simulink model "UAV_2010_simulink_model_run"  (R2022b)
settings: Solver=VariableStepAuto  StartTime=0.0  StopTime=t_end  RelTol=1e-3
values from neighbouring files (symbols this model uses):
  alt0 = 500    [Run_nonlinear_2010UAV_sim.m]
  lat0 = deg2rad(63.9963)    [Run_nonlinear_2010UAV_sim.m]
  long0 = deg2rad(-22.6237)    [Run_nonlinear_2010UAV_sim.m]
  windseed = [randi([0 4000], 1, 4)]    [Run_nonlinear_2010UAV_sim.m]
  X_init = X_trim_point    [Run_nonlinear_2010UAV_sim.m]
undefined symbols (not defined in the file or in its folder): F, Light, MIL, Receive, Send
libraries: aerolibfltsims x4, aerolibwind2 x2, aerolibatmos2 x1
settings Model: Creator=aaron  LastModifiedBy=aaron
settings DataIOCC: SaveFormat=StructureWithTime
settings DebuggingCC: UnderSpecifiedDimensionMsg=warning

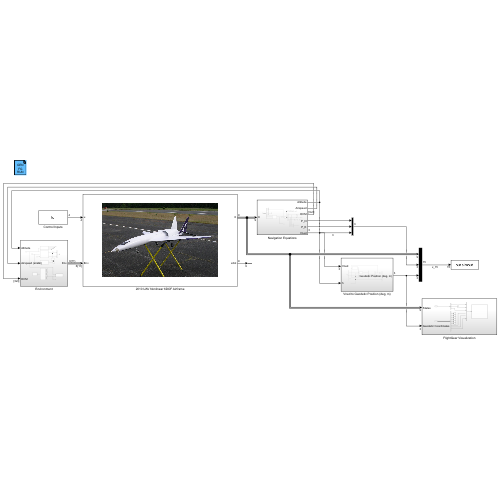
[thumbnail: Simulink's stored preview of the top-level diagram]
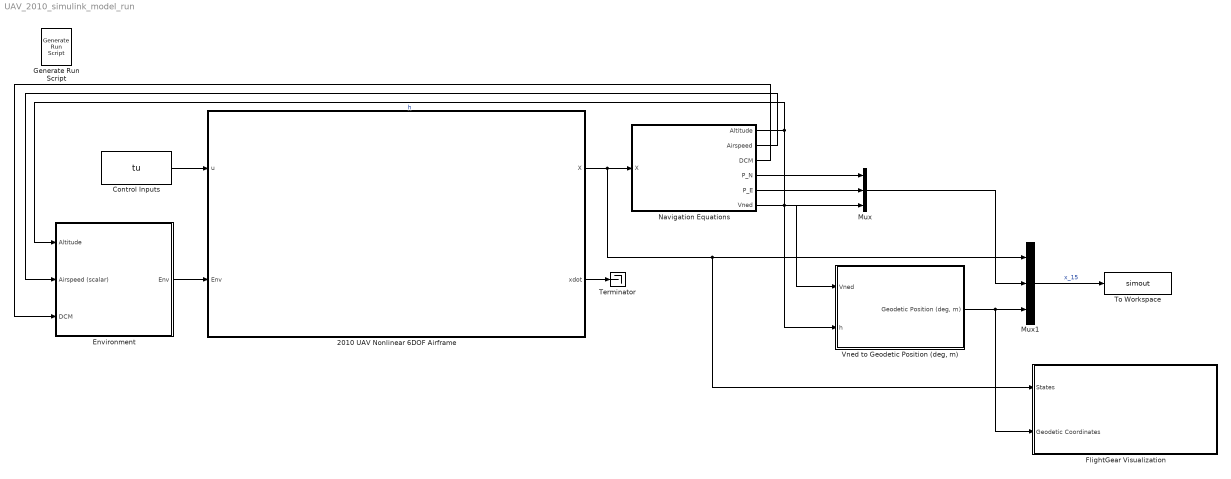
== system UAV_2010_simulink_model_run ==
  2010 UAV Nonlinear 6DOF Airframe : Subsystem
      mask Display: image('$imagefile'); % Use "Edit Image" on toolstrip to change.
  Control Inputs : FromWorkspace  VariableName=tu
  Environment : Subsystem
  FlightGear Visualization : Subsystem
  Generate Run Script : aerolibfltsims/Generate Run Script  Architecture=Default  dataFlow=Send-Receive  GeometryModelName=c172p  AirportId=KSFO  RunwayId=10L  InitialAltitude=7224  InitialHeading=113  OffsetDistance=4.72  OffsetAzimuth=0  InstallScenery=off  DisableShaders=on  OriginAddress=127.0.0.1  DestinationPort=5502  OriginPort=5505  LocalAddress=127.0.0.1  OutputFileName=fg_simulink_2010UAV.bat  FlightGearBaseDirectory=C:\Program Files\FlightGear 2020.3
  Mux : Mux  Inputs=3
  Mux1 : Mux  Inputs=[9 3 3]
  Navigation Equations : Subsystem
  Terminator : Terminator
  To Workspace : ToWorkspace  VariableName=simout  SaveFormat=Structure With Time  SampleTime=-1
  "Vned to Geodetic Position (deg, m)" : Subsystem
  wires:
  Control Inputs/1 -> 2010 UAV Nonlinear 6DOF Airframe/1(u)
  2010 UAV Nonlinear 6DOF Airframe/2(xdot) -> Terminator/1
  2010 UAV Nonlinear 6DOF Airframe/1(X) -> Navigation Equations/1(X), FlightGear Visualization/1(States), Mux1/1
  Navigation Equations/4(P_N) -> Mux/1
  Navigation Equations/5(P_E) -> Mux/2
  Navigation Equations/1(Altitude) -> Mux/3, "Vned to Geodetic Position (deg, m)"/2(h), Environment/1(Altitude)  "h"
  Navigation Equations/3(DCM) -> Environment/3(DCM)
  Mux/1 -> Mux1/2
  Mux1/1 -> To Workspace/1  "x_15"
  Navigation Equations/2(Airspeed) -> Environment/2(Airspeed (scalar))
  Navigation Equations/6(Vned) -> "Vned to Geodetic Position (deg, m)"/1(Vned)
  "Vned to Geodetic Position (deg, m)"/1("Geodetic Position (deg, m)") -> FlightGear Visualization/2(Geodetic Coordinates), Mux1/3
  Environment/1(Env) -> 2010 UAV Nonlinear 6DOF Airframe/2(Env)

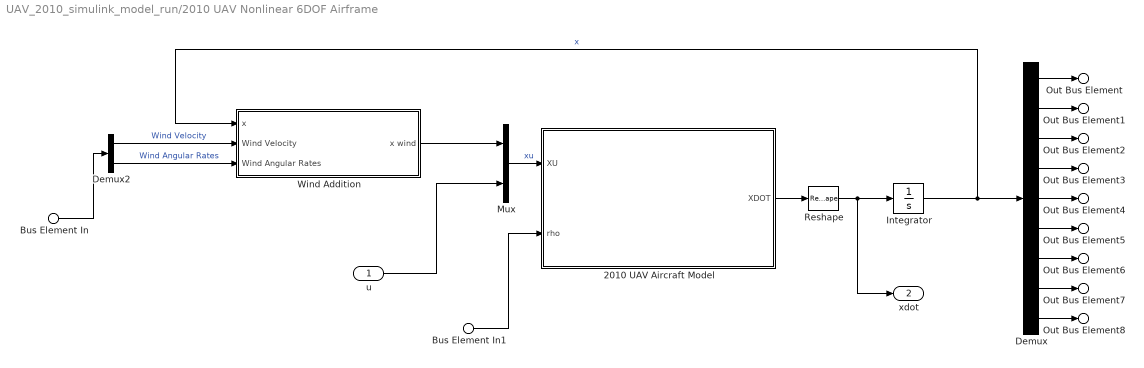
== system UAV_2010_simulink_model_run/2010 UAV Nonlinear 6DOF Airframe ==
  u : Inport
  Bus Element In : Inport  Port=2  PortName=Env  Element=Wind
  Bus Element In1 : Inport  Port=2  PortName=Env  Element=AirDensity
  2010 UAV Aircraft Model : MATLAB Function  TreatAsAtomicUnit=on
  Demux : Demux  Outputs=9
  Demux2 : Demux  Outputs=[3 3]
  Integrator : Integrator  InitialCondition=X_init
  Mux : Mux  Inputs=[9 4]
  Reshape : Reshape
  Wind Addition : Subsystem
  Out Bus Element : Outport  PortName=X  Element=u
  Out Bus Element1 : Outport  PortName=X  Element=v
  Out Bus Element2 : Outport  PortName=X  Element=w
  Out Bus Element3 : Outport  PortName=X  Element=p
  Out Bus Element4 : Outport  PortName=X  Element=q
  Out Bus Element5 : Outport  PortName=X  Element=r
  Out Bus Element6 : Outport  PortName=X  Element=phi
  Out Bus Element7 : Outport  PortName=X  Element=theta
  Out Bus Element8 : Outport  PortName=X  Element=psi
  xdot : Outport  Port=2
  wires:
  u/1 -> Mux/2
  Mux/1 -> 2010 UAV Aircraft Model/1(XU)  "xu"
  2010 UAV Aircraft Model/1(XDOT) -> Reshape/1
  Reshape/1 -> Integrator/1, xdot/1
  Integrator/1 -> Wind Addition/1(x), Demux/1  "x"
  Demux/1 -> Out Bus Element/1
  Demux/2 -> Out Bus Element1/1
  Demux/3 -> Out Bus Element2/1
  Demux/4 -> Out Bus Element3/1
  Demux/5 -> Out Bus Element4/1
  Demux/6 -> Out Bus Element5/1
  Demux/7 -> Out Bus Element6/1
  Demux/8 -> Out Bus Element7/1
  Demux/9 -> Out Bus Element8/1
  Demux2/1 -> Wind Addition/2(Wind Velocity)  "Wind Velocity"
  Demux2/2 -> Wind Addition/3(Wind Angular Rates)  "Wind Angular Rates"
  Wind Addition/1(x wind) -> Mux/1
  Bus Element In/1 -> Demux2/1
  Bus Element In1/1 -> 2010 UAV Aircraft Model/2(rho)

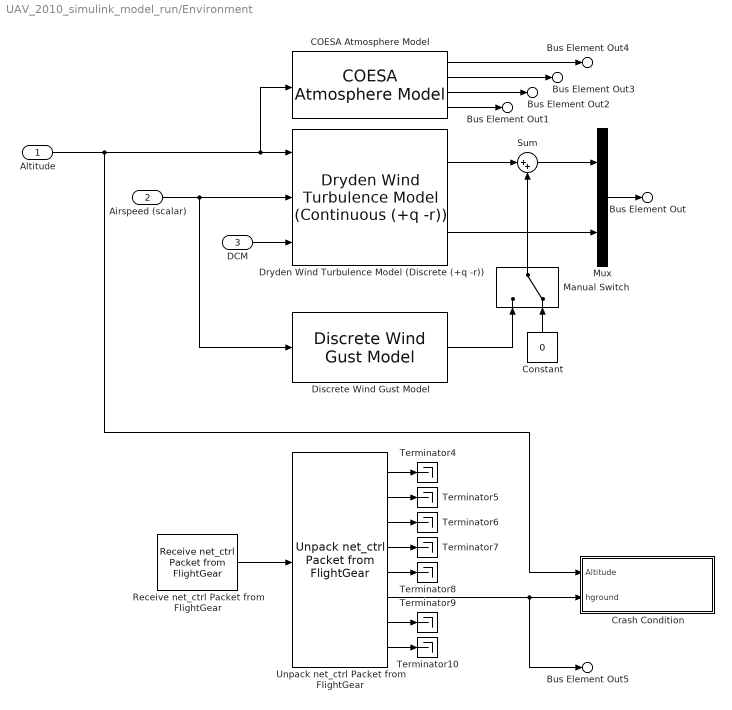
== system UAV_2010_simulink_model_run/Environment ==
  Altitude : Inport
  Airspeed (scalar) : Inport  Port=2
  DCM : Inport  Port=3
  COESA Atmosphere Model : aerolibatmos2/COESA Atmosphere Model  units=Metric (MKS)  spec=1976 COESA-extended U.S. Standard Atmosphere  model=Profile  profile_var=High temperature  profile_percent=1%  profile_alt=5 km (16404 ft)  envelope_var=High temperature  envelope_percent=1%  action=Warning
  Constant : Constant  Value=0
  Crash Condition : Subsystem
  Discrete Wind Gust Model : aerolibwind2/Discrete Wind Gust Model  units=Metric (MKS)  Gx=on  Gy=on  Gz=on  t_0=14  d_m=[120 120 80]  v_m=[3.5 3.5 3.0]
  Dryden Wind Turbulence Model (Discrete (+q -r)) : aerolibwind2/Dryden Wind Turbulence Model  (Continuous (+q -r))  units=Metric (MKS)  spec=MIL-F-8785C  model=Continuous Dryden (+q -r)  W20=3  Wdeg=0  TurbProb=10^-2 - Light  L_high=533.4  Wingspan=1.8657850784  ts=0.1  Seed=windseed  T_on=on
      settings: LibrarySourceBlock=|
      | aerolibwind2/Dryden Wind Turbulence Model
      | (Discrete (+q -r))
  Manual Switch : ManualSwitch  CurrentSetting=0
  Mux : Mux  Inputs=2
  Receive net_ctrl Packet from FlightGear : aerolibfltsims/Receive net_ctrl Packet from FlightGear  FlightGearVersion=v2019.1  ReceiveAddress=127.0.0.1  ReceivePort=5505  ReceiveWidth=744  varLen=off  SampleTime=1/30  packetFlag=off
  Sum : Sum  Inputs=|++
  Terminator{4..10} (7 alike) : Terminator
  Unpack net_ctrl Packet from FlightGear : aerolibfltsims/Unpack net_ctrl Packet from FlightGear  FlightGearVersion=v2019.1  ShowControlSurfacePositionOutputs=off  ShowEngineFuelOutputs=off  ShowLandingGearOutputs=off  ShowAvionicOutputs=off  ShowEnvironmentOutputs=on  SampleTime=1/30  packetVersion=27
  Bus Element Out : Outport  PortName=Env  Element=Wind
  Bus Element Out1 : Outport  PortName=Env  Element=AirDensity
  Bus Element Out2 : Outport  PortName=Env  Element=Air Pressure
  Bus Element Out3 : Outport  PortName=Env  Element=Speed of Sound
  Bus Element Out4 : Outport  PortName=Env  Element=Temperature
  Bus Element Out5 : Outport  PortName=Env  Element=hground
  wires:
  COESA Atmosphere Model/1 -> Bus Element Out4/1
  COESA Atmosphere Model/2 -> Bus Element Out3/1
  COESA Atmosphere Model/3 -> Bus Element Out2/1
  COESA Atmosphere Model/4 -> Bus Element Out1/1
  Dryden Wind Turbulence Model (Discrete (+q -r))/2 -> Mux/2
  Mux/1 -> Bus Element Out/1
  Unpack net_ctrl Packet from FlightGear/5 -> Terminator8/1
  Unpack net_ctrl Packet from FlightGear/8 -> Terminator10/1
  Unpack net_ctrl Packet from FlightGear/2 -> Terminator5/1
  Unpack net_ctrl Packet from FlightGear/6 -> Bus Element Out5/1, Crash Condition/2(hground)
  Unpack net_ctrl Packet from FlightGear/7 -> Terminator9/1
  Unpack net_ctrl Packet from FlightGear/1 -> Terminator4/1
  Unpack net_ctrl Packet from FlightGear/4 -> Terminator7/1
  Receive net_ctrl Packet from FlightGear/1 -> Unpack net_ctrl Packet from FlightGear/1
  Unpack net_ctrl Packet from FlightGear/3 -> Terminator6/1
  Altitude/1 -> Crash Condition/1(Altitude), COESA Atmosphere Model/1, Dryden Wind Turbulence Model (Discrete (+q -r))/1
  Airspeed (scalar)/1 -> Discrete Wind Gust Model/1, Dryden Wind Turbulence Model (Discrete (+q -r))/2
  DCM/1 -> Dryden Wind Turbulence Model (Discrete (+q -r))/3
  Dryden Wind Turbulence Model (Discrete (+q -r))/1 -> Sum/1
  Sum/1 -> Mux/1
  Manual Switch/1 -> Sum/2
  Discrete Wind Gust Model/1 -> Manual Switch/1
  Constant/1 -> Manual Switch/2

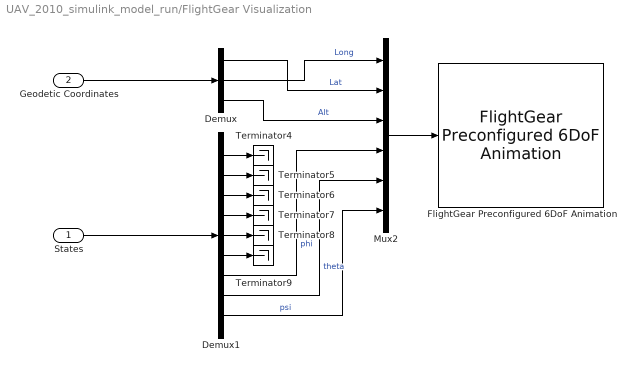
== system UAV_2010_simulink_model_run/FlightGear Visualization ==
  States : Inport
  Geodetic Coordinates : Inport  Port=2
  Demux : Demux  Outputs=[1 1 1]
  Demux1 : Demux  Outputs=[1 1 1 1 1 1 1 1 1]
  FlightGear Preconfigured 6DoF Animation : aerolibfltsims/FlightGear Preconfigured 6DoF Animation  xFlightGearVersion=v2019.1  DestinationIpAddress=127.0.0.1  DestinationPort=5502  SampleTime=1/30  packetVersion=24
  Mux2 : Mux  Inputs=[1 1 1 1 1 1]
  Terminator{4..9} (6 alike) : Terminator
  wires:
  States/1 -> Demux1/1
  Demux1/1 -> Terminator4/1
  Demux1/6 -> Terminator9/1
  Demux/2 -> Mux2/1  "Long"
  Demux/3 -> Mux2/3  "Alt"
  Demux1/3 -> Terminator6/1
  Demux1/9 -> Mux2/6  "psi"
  Demux1/4 -> Terminator7/1
  Demux1/7 -> Mux2/4  "phi"
  Demux1/2 -> Terminator5/1
  Demux1/5 -> Terminator8/1
  Mux2/1 -> FlightGear Preconfigured 6DoF Animation/1
  Demux1/8 -> Mux2/5  "theta"
  Demux/1 -> Mux2/2  "Lat"
  Geodetic Coordinates/1 -> Demux/1

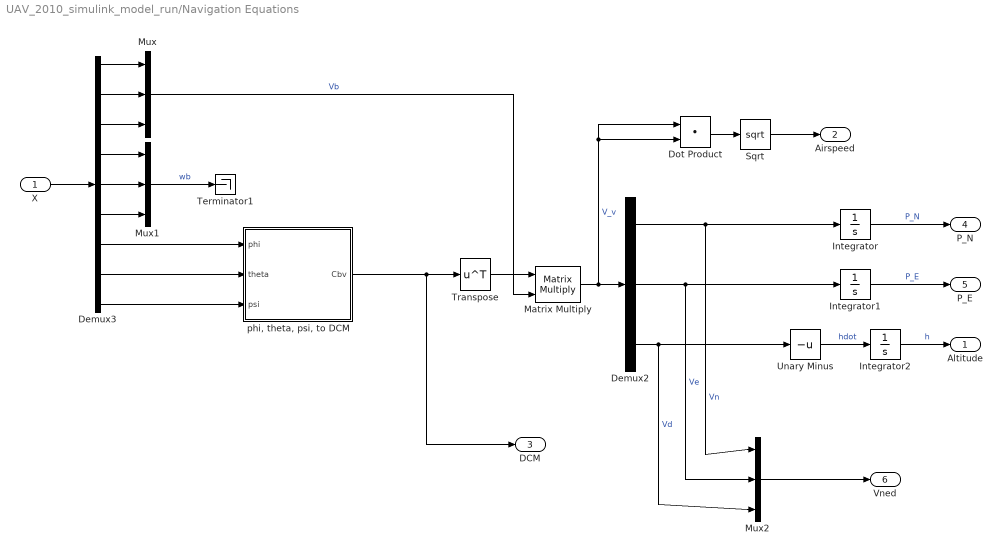
== system UAV_2010_simulink_model_run/Navigation Equations ==
  X : Inport
  Demux2 : Demux  Outputs=3
  Demux3 : Demux  Outputs=9
  Dot Product : DotProduct  OutDataTypeStr=Inherit: Inherit via internal rule
  Integrator : Integrator
  Integrator1 : Integrator
  Integrator2 : Integrator  InitialCondition=alt0
  Matrix Multiply : Product  Multiplication=Matrix(*)
  Mux : Mux  Inputs=3
  Mux1 : Mux  Inputs=3
  Mux2 : Mux  Inputs=[1 1 1]
  Sqrt : Sqrt
  Terminator1 : Terminator
  Transpose : Math  Operator=transpose
  Unary Minus : UnaryMinus
  "phi, theta, psi, to DCM" : MATLAB Function  TreatAsAtomicUnit=on
  Altitude : Outport
  Airspeed : Outport  Port=2
  DCM : Outport  Port=3
  P_N : Outport  Port=4
  P_E : Outport  Port=5
  Vned : Outport  Port=6
  wires:
  Integrator1/1 -> P_E/1  "P_E"
  Demux3/8 -> "phi, theta, psi, to DCM"/2(theta)
  Integrator/1 -> P_N/1  "P_N"
  Matrix Multiply/1 -> Dot Product/1, Dot Product/2, Demux2/1  "V_v"
  Transpose/1 -> Matrix Multiply/1
  Mux/1 -> Matrix Multiply/2  "Vb"
  Mux1/1 -> Terminator1/1  "wb"
  Demux3/7 -> "phi, theta, psi, to DCM"/1(phi)
  Integrator2/1 -> Altitude/1  "h"
  Demux2/2 -> Mux2/2, Integrator1/1  "Ve"
  Demux2/1 -> Mux2/1, Integrator/1  "Vn"
  Demux3/9 -> "phi, theta, psi, to DCM"/3(psi)
  "phi, theta, psi, to DCM"/1(Cbv) -> Transpose/1, DCM/1
  Unary Minus/1 -> Integrator2/1  "hdot"
  Demux2/3 -> Unary Minus/1, Mux2/3  "Vd"
  X/1 -> Demux3/1
  Demux3/1 -> Mux/1
  Demux3/2 -> Mux/2
  Demux3/3 -> Mux/3
  Demux3/4 -> Mux1/1
  Demux3/5 -> Mux1/2
  Demux3/6 -> Mux1/3
  Dot Product/1 -> Sqrt/1
  Sqrt/1 -> Airspeed/1
  Mux2/1 -> Vned/1

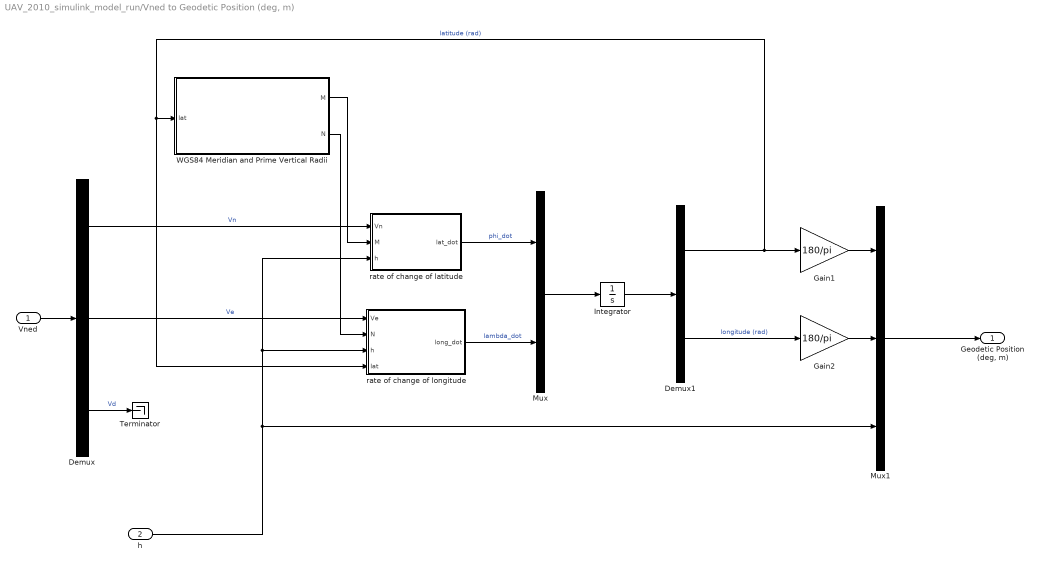
== system UAV_2010_simulink_model_run/Vned to Geodetic Position (deg, m) ==
  Vned : Inport
  h : Inport  Port=2
  Demux : Demux  Outputs=[1 1 1]
  Demux1 : Demux  Outputs=[1 1]
  Gain1 : Gain  Gain=180/pi
  Gain2 : Gain  Gain=180/pi
  Integrator : Integrator  InitialCondition=[lat0 long0]
  Mux : Mux  Inputs=[1 1]
  Mux1 : Mux  Inputs=[1 1 1]
  Terminator : Terminator
  WGS84 Meridian and Prime Vertical Radii : MATLAB Function  TreatAsAtomicUnit=on
  rate of change of latitude : MATLAB Function  TreatAsAtomicUnit=on
  rate of change of longitude : MATLAB Function  TreatAsAtomicUnit=on
  "Geodetic Position (deg, m)" : Outport
  wires:
  Vned/1 -> Demux/1
  Demux/1 -> rate of change of latitude/1(Vn)  "Vn"
  Demux/2 -> rate of change of longitude/1(Ve)  "Ve"
  Mux/1 -> Integrator/1
  rate of change of latitude/1(lat_dot) -> Mux/1  "phi_dot"
  rate of change of longitude/1(long_dot) -> Mux/2  "lambda_dot"
  Integrator/1 -> Demux1/1
  Demux1/2 -> Gain2/1  "longitude (rad)"
  Demux1/1 -> Gain1/1, rate of change of longitude/4(lat), WGS84 Meridian and Prime Vertical Radii/1(lat)  "latitude (rad)"
  Mux1/1 -> "Geodetic Position (deg, m)"/1
  WGS84 Meridian and Prime Vertical Radii/1(M) -> rate of change of latitude/2(M)
  WGS84 Meridian and Prime Vertical Radii/2(N) -> rate of change of longitude/2(N)
  Gain1/1 -> Mux1/1
  Gain2/1 -> Mux1/2
  Demux/3 -> Terminator/1  "Vd"
  h/1 -> Mux1/3, rate of change of latitude/3(h), rate of change of longitude/3(h)

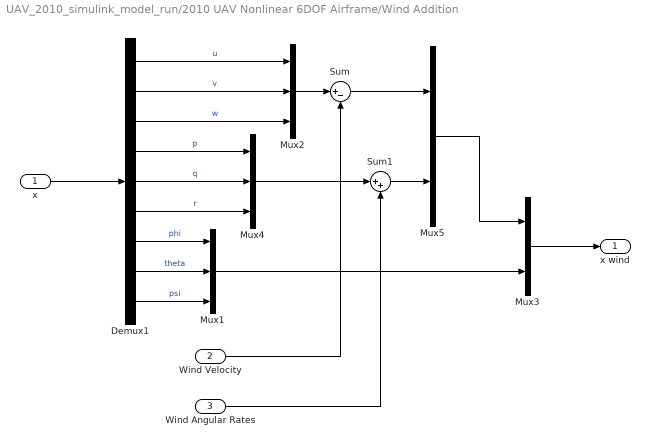
== system UAV_2010_simulink_model_run/2010 UAV Nonlinear 6DOF Airframe/Wind Addition ==
  x : Inport
  Wind Velocity : Inport  Port=2
  Wind Angular Rates : Inport  Port=3
  Demux1 : Demux  Outputs=[1 1 1 1 1 1 1 1 1]
  Mux1 : Mux  Inputs=[1 1 1]
  Mux2 : Mux  Inputs=[1 1 1]
  Mux3 : Mux  Inputs=[6, 3]
  Mux4 : Mux  Inputs=[1 1 1]
  Mux5 : Mux  Inputs=[3 3]
  Sum : Sum  Inputs=|+-
  Sum1 : Sum  Inputs=|++
  x wind : Outport
  wires:
  Sum/1 -> Mux5/1
  Demux1/1 -> Mux2/1  "u"
  Demux1/3 -> Mux2/3  "w"
  Mux4/1 -> Sum1/1
  Demux1/4 -> Mux4/1  "p"
  Wind Angular Rates/1 -> Sum1/2
  Mux2/1 -> Sum/1
  Demux1/7 -> Mux1/1  "phi"
  Demux1/6 -> Mux4/3  "r"
  Demux1/5 -> Mux4/2  "q"
  Mux1/1 -> Mux3/2
  Demux1/2 -> Mux2/2  "v"
  Demux1/9 -> Mux1/3  "psi"
  Sum1/1 -> Mux5/2
  Mux5/1 -> Mux3/1
  Demux1/8 -> Mux1/2  "theta"
  Wind Velocity/1 -> Sum/2
  x/1 -> Demux1/1
  Mux3/1 -> x wind/1

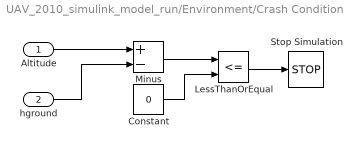
== system UAV_2010_simulink_model_run/Environment/Crash Condition ==
  Altitude : Inport
  hground : Inport  Port=2
  Constant : Constant  Value=0
  LessThanOrEqual : RelationalOperator  Operator=<=  OutDataTypeStr=boolean  RndMeth=Simplest  InputSameDT=off
  Minus : Sum  Inputs=+-
  Stop Simulation : Stop
  wires:
  Minus/1 -> LessThanOrEqual/1
  Altitude/1 -> Minus/1
  LessThanOrEqual/1 -> Stop Simulation/1
  Constant/1 -> LessThanOrEqual/2
  hground/1 -> Minus/2

== matlab function UAV_2010_simulink_model_run/Vned to Geodetic Position (deg, m)/WGS84 Meridian and Prime Vertical Radii ==
  data: lat input; M output; N output
function [M, N] = meridian_curvature(lat)

a = 6378137.0;
e = 0.081819190842622;

M = a*(1-e^2)/(1 - e^2*sin(lat)^2)^(3/2);
N = a/(1 - e^2*sin(lat)^2)^(1/2);

== matlab function UAV_2010_simulink_model_run/Navigation Equations/phi, theta, psi, to DCM ==
  data: phi input; Cbv output; theta input; psi input
function Cbv = calc_Cbv(phi, theta, psi)

C1v = [ cos(psi) sin(psi)  0
       -sin(psi) cos(psi)  0
        0        0         1];

C21 = [cos(theta)  0  -sin(theta)
       0           1   0
       sin(theta)  0   cos(theta)];

Cb2 = [1  0        0
       0  cos(phi) sin(phi)
       0 -sin(phi) cos(phi)];

Cbv = Cb2*C21*C1v;

== matlab function UAV_2010_simulink_model_run/2010 UAV Nonlinear 6DOF Airframe/2010 UAV Aircraft Model ==
  data: XU input; XDOT output; rho input
function XDOT  = UAV_2010_model_for_Simulink(XU, rho)

%------------------STATE AND CONTROL VECTOR--------------------------------
% Extract state vector
x1 = XU(1); % u
x2 = XU(2); % v
x3 = XU(3); % w
x4 = XU(4); % p
x5 = XU(5); % q
x6 = XU(6); % r
x7 = XU(7); % phi
x8 = XU(8); % theta
x9 = XU(9); % psi

U = XU(10:13);

u1 = U(1); %d_A (aileron)
u2 = U(2); %d_T (stabilizer)
u3 = U(3); %d_R (rudder)
u4 = U(4); %d_th1 (throttle 1)

%---------------------CONSTANTS--------------------------------------------
% Nominal vehicle constants
m = 16.55612;            % Aircraft total mass (kg)

cbar = 0.7020814;        % Mean Aerodynamic Chord (m)
S = 1.309933;            % Wing planform area

Xcg = 0.2*cbar;          % x position of CoG in Fm (m)
Ycg = 0*cbar;            % y position of CoG in Fm (m)
Zcg = -0.10*cbar;        % z position of CoG in Fm (m)

% Engine constants
Xapt1 = -0.3556;         % x position of engine 1 force in Fm (m)
Yapt1 = 0;               % x position of engine 1 force in Fm (m)
Zapt1 = -0.0508;         % x position of engine 1 force in Fm (m)

% Other constants
g = 9.81;                % grav constant

%---------------------1. CONTROL LIMITS/SATURATION-------------------------


%---------------------2. INTERMEDIATE VARIABLES----------------------------
% Calculate airspeed
Va = sqrt(x1^2 + x2^2 + x3^2);

% Calculate alpha and beta
alpha = atan2(x3,x1)*180/pi;
beta = asin(x2/Va)*180/pi;

% Calculate dynamic pressure
Q = 0.5*rho*Va^2;

% Define vectors wbe_b and V_b
wbe_b = [x4;x5;x6];
V_b = [x1;x2;x3];

%---------------------3. AERODYNAMIC FORCE COEFFICIENTS--------------------
% Calculate the CL_wb

CL_noElev = -0.00002271*alpha^3 - 0.0002302*alpha^2 + 0.06565*alpha + 0.03959; % CL

CL_elevEffect = (-0.00001250958*alpha^3 + 0.000007639437*alpha^2 + 0.000286478898*alpha + 0.625574419317)*u2; % elevator effect on lift

% Total lift force coefficient
CL = CL_noElev + CL_elevEffect;  

% Total drag force
CD = 0.000857*alpha^2 - 0.0004961*alpha + 0.0217;   % Curve fit of CD vs alpha

% % Total side force
if beta > 30.857                                    % piecewise parametrization of side force coefficient
    CY = 0.004409*beta -0.1694;
elseif beta <= 30.857 && beta >= -30.857
    CY = -0.001126*beta + 0.001396;
else
    CY = 0.004409*beta -0.1694;
end
%---------------------4. DIMENSIONAL AERODYNAMIC FORCES--------------------
% Calculate the actual dimensional forces in F_s (stability axis)
FA_s = [-CD*Q*S;
        CY*Q*S;
        -CL*Q*S];

rad = pi/180;

C_bs = [cos(alpha*rad) 0 -sin(alpha*rad);
        0 1 0;
        sin(alpha*rad) 0 cos(alpha*rad)];

FA_b = C_bs*FA_s;

%---------------------5. AERODYNAMIC MOMENT COEFFICIENT ABOUT CG --------------------
% Calculate CM = [Cl;Cm;Cn] about aerodynamic center in Fb

if beta > -17.409 && beta < 17.409                       % piecewise parameterization of CR
    eta11 = -0.0001058*(beta) + 0.0002933;
elseif beta <= -17.409
    eta11 = 0.0005473*beta + 0.01108;
else 
    eta11 = 0.0005473*beta -0.01108;
end

eta21 = CMBA_lookup_table_2010_UAV(alpha, beta);           % CM lookup table
eta31 = CNBA_lookup_2010_UAV(beta);                        % CN lookup table

CMcg_b = [eta11 - 0.02864*u1 + dCRBA_dRudder(u3, alpha);       % all moments about CG in body axis including control surface effectiveness
          eta21 + dCMSA_dElevator(u2, alpha, beta);
          eta31 + dCNBA_dRudder(alpha, u3)];

%---------------------6. AERODYNAMIC MOMENT ABOUT CG --------------------
% Normalize to an aerodynamic moment
MAcg_b = CMcg_b*Q*S*cbar;

% %---------------------7. AERODYNAMIC  COEFFICIENT ABOUT CG --------------------------
% rcg_b = [Xcg;Ycg;Zcg];
% rac_b = [Xac;Yac;Zac];
% MAcg_b = MAac_b + cross(FA_b,rcg_b - rac_b);

%---------------------8. ENGINE FORCE AND MOMENT ------------------------------------
% effect of engine. First, calculate thrust of engine
% engine_coeffs = [1.012e-09, -5.527e-05, 1.044];
% 
% RPM = 158000*u4;
% if u4 > 1
%     RPM = 158000;
% end
% if RPM >= 0
%     F1 = (engine_coeffs(1)*RPM^2 + engine_coeffs(2)*RPM + engine_coeffs(3))*4.44822;
% else
%     F1 = 0;
% end

F1 = u4*m*g;

% assuming engine thrust is aligned with Fb, we have
FE1_b = [F1;0;0];
FE_b = FE1_b;

% engine moment due to offset of engine thrust from CoG
mew1 = [Xcg - Xapt1;
        Yapt1 - Ycg;
        Zcg - Zapt1];

MEcg1_b = cross(mew1,FE1_b);

MEcg_b = MEcg1_b;

%---------------------9. GRAVITY EFFECTS ------------------------------------
% Calculate gravitational forces in the body frame. This causes no moment
% about CoG
g_b = [-g*sin(x8);
        g*cos(x8)*sin(x7);
        g*cos(x8)*cos(x7)];

Fg_b = m*g_b;

%---------------------10. GRAVITY EFFECTS ------------------------------------
% Inertia matrix
Ib = [1.1619 0 -0.0607;
        0 5.6276 0;
        -0.0607 0 6.1040];

% Inverse of inertia matrix
% symmetric about xz plane
invIb =    [0.861106618696125	0	                0.00856310153257778
            0	                0.177695642902836	0
            0.00856310153257778	0	                0.163912152729854];

% Form R_b (all forces in Fb) and calculate udot, vdot, wdot
F_b = Fg_b + FE_b + FA_b;
x1to3dot = (1/m)*F_b - cross(wbe_b,V_b);

% Form Mcg_b (all moments about CoG in Fb) and calculate pdot, qdot, rdot
Mcg_b = MAcg_b+MEcg_b;
x4to6dot = invIb*(Mcg_b - cross(wbe_b,Ib*wbe_b));

% Calculate phidot, thetadot, psidot
H_phi = [1 sin(x7)*tan(x8) cos(x7)*tan(x8);
         0 cos(x7) -sin(x7);
         0 sin(x7)/cos(x8) cos(x7)/cos(x8)];

x7to9dot = H_phi*wbe_b;

% Place in first order form
XDOT = [x1to3dot; 
        x4to6dot; 
        x7to9dot];

%     function tan = atan2_0_pi(y,x)
%         if x == 0
%             if y == 0
%                 tan = 0;
%             elseif y > 0
%                 tan = pi/2;
%             else
%                 tan = 3*pi/3;
%             end
%         elseif x > 0
%             if y >= 0
%                 tan = atan(y/x);
%             else
%                 tan = atan(y/x) + 2*pi;
%             end
%         elseif x < 0
%             if y == 0
%                 tan = pi;
%             else
%                 tan = atan(y/x) + pi;
%             end
%         end
%     end

end

== matlab function UAV_2010_simulink_model_run/Vned to Geodetic Position (deg, m)/rate of change of latitude ==
  data: Vn input; lat_dot output; M input; h input
function lat_dot = latitude_rate(Vn, M, h)

lat_dot = Vn/(M+h);

== matlab function UAV_2010_simulink_model_run/Vned to Geodetic Position (deg, m)/rate of change of longitude ==
  data: Ve input; long_dot output; N input; h input; lat input
function long_dot = longitude_rate(Ve, N, h, lat)

long_dot = Ve/((N+h)*cos(lat));
